simulink model "P7_simulink"  (R2023a)
settings: Solver=VariableStepAuto  StartTime=0.0  StopTime=8  RelTol=1e-3
values from neighbouring files (symbols this model uses):
  C1 = 1e-6    (= 1e-06)    [P7_OpAmp.m]
  C2 = 1e-6    (= 1e-06)    [P7_OpAmp.m]
  R1 = 5e6    (= 5000000)    [P7_OpAmp.m]
  R2 = 5e6    (= 5000000)    [P7_OpAmp.m]
  R3 = 5e6    (= 5000000)    [P7_OpAmp.m]
settings Model: Creator=karen  LastModifiedBy=karen

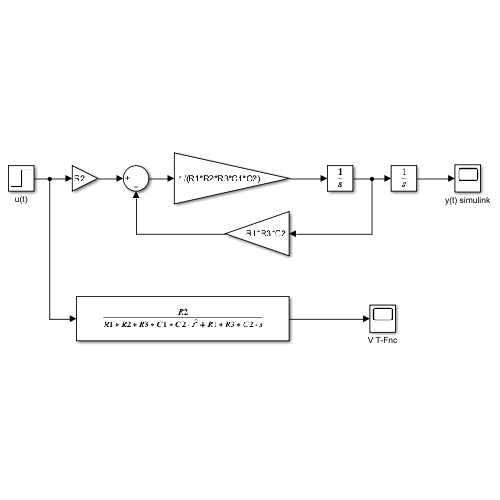
[thumbnail: Simulink's stored preview of the top-level diagram]
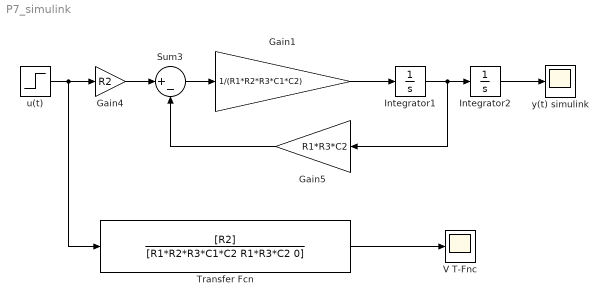
== system P7_simulink ==
  Gain1 : Gain  Gain=1/(R1*R2*R3*C1*C2)
  Gain4 : Gain  Gain=R2
  Gain5 : Gain  Gain=R1*R3*C2
  Integrator1 : Integrator
  Integrator2 : Integrator
  Sum3 : Sum  Inputs=|+-
  Transfer Fcn : TransferFcn  Numerator=[R2]  Denominator=[R1*R2*R3*C1*C2 R1*R3*C2 0]
  V T-Fnc : Scope
  u(t) : Step  Time=0  After=5  SampleTime=0
  y(t) simulink : Scope
  wires:
  Gain1/1 -> Integrator1/1
  Sum3/1 -> Gain1/1
  Integrator2/1 -> y(t) simulink/1
  Gain5/1 -> Sum3/2
  Gain4/1 -> Sum3/1
  Integrator1/1 -> Gain5/1, Integrator2/1
  u(t)/1 -> Transfer Fcn/1, Gain4/1
  Transfer Fcn/1 -> V T-Fnc/1
